simulink model "tanks2"  (R2025b)
settings: Solver=VariableStepAuto  StartTime=0.0  StopTime=10.0  RelTol=1e-3
model workspace (MAT data in the model file):
  sine_amp = 0.2
values from neighbouring files (symbols this model uses):
  a = 0.2    [tanks.m]
  omega1 = 8    [tanks.m]
  omega2 = 5    [tanks.m]
  qbar1 = 1.5    [tanks.m]
  qbar2 = 0.5    [tanks.m]
settings Model: Creator=jbrouill  LastModifiedBy=seby
settings SolverCC: AlgebraicLoopSolver=TrustRegion
settings DataIOCC: Refine=10
settings DebuggingCC: UnconnectedInputMsg=warning  UnconnectedOutputMsg=warning  UnconnectedLineMsg=warning
settings ModelReferenceCC: EnableRefExpFcnMdlSchedulingChecks=on
settings RTWCC: GPUComputeCapability=3.5

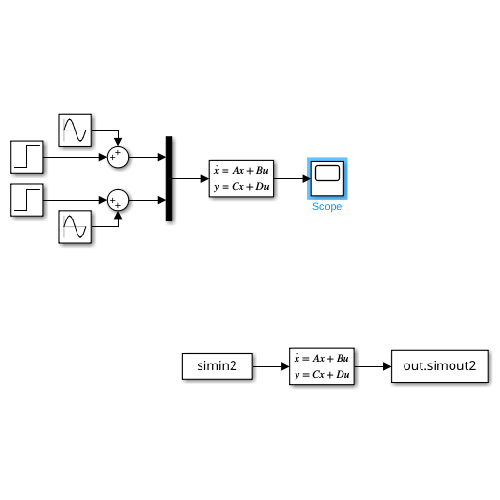
[thumbnail: Simulink's stored preview of the top-level diagram]
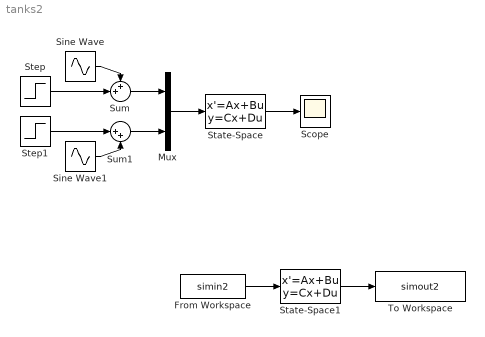
== system tanks2 ==
  From Workspace : FromWorkspace  VariableName=simin2
  Mux : Mux  Inputs=2
  Scope : Scope
      settings: ActiveDisplayYMinimum=-1.8204532385186565  ActiveDisplayYMaximum=3.8303368545726895
  Sine Wave : Sin  Amplitude=a  Frequency=omega1  SampleTime=0
  Sine Wave1 : Sin  Amplitude=a  Frequency=omega2  SampleTime=0
  State-Space : StateSpace  A=[-3 0; 3 -5]  B=[1 0 ; 0 1]  C=[3 0 ; 0 5]  D=zeros(2,2)  InitialCondition=[0.1 ; 0.1]
  State-Space1 : StateSpace  A=[-3 0; 3 -5]  B=[1 0 ; 0 1]  C=[3 0 ; 0 5]  D=zeros(2,2)  InitialCondition=[0.1 ; 0.1]
  Step : Step  Time=0  After=qbar1  SampleTime=0
  Step1 : Step  Time=0  After=qbar2  SampleTime=0
  Sum : Sum  Inputs=++|
  Sum1 : Sum  Inputs=|++
  To Workspace : ToWorkspace  VariableName=simout2  SaveFormat=Timeseries  SampleTime=-1
  wires:
  Step/1 -> Sum/2
  State-Space/1 -> Scope/1
  Sine Wave/1 -> Sum/1
  State-Space1/1 -> To Workspace/1
  From Workspace/1 -> State-Space1/1
  Sum/1 -> Mux/1
  Sum1/1 -> Mux/2
  Step1/1 -> Sum1/1
  Sine Wave1/1 -> Sum1/2
  Mux/1 -> State-Space/1
